simulink model "ROS2"  (R2018b)
settings: Solver=ode5  StartTime=0.0  StopTime=10  FixedStep=0.001  RelTol=1e-3  EnableMultiTasking=on
InitFcn:
  | clear;
  | clc;
  | close all;
  | L1=[1 0 0 -1;-1 1 0 0;0 -1 1 0;0 0 -1 1];
  | 
  | I2=eye(2);
  | LK1=kron(L1,I2);
  | LK1=-LK1;
  | %E matrix
  | E=eye(8);
  | x0=[0 0 0 0 0 0 0 0];
  | x02=[x0(1) x0(3) x0(5) x0(7) x0(2) x0(4) x0(6) x0(8)];
  | x0=x0';
  | 
  | v0=[1 1 2 1 1 1 1 1]';
  | xd=[20 20 30 20 30 10 20 10];
  | 
  | PID=[10,1,0,100];
  | 
  | M=[1 1;1 -1];
StopFcn:
  | figure
  | x_trajectory_1=trajectory(:,1);
  | y_trajectory_1=trajectory(:,5);
  | x_trajectory_2=trajectory(:,2);
  | y_trajectory_2=trajectory(:,6);
  | x_trajectory_3=trajectory(:,3);
  | y_trajectory_3=trajectory(:,7);
  | x_trajectory_4=trajectory(:,4);
  | y_trajectory_4=trajectory(:,8);
  | 
  | plot(x_trajectory_1,y_trajectory_1,x_trajectory_2,y_trajectory_2,x_trajectory_3,y_trajectory_3,x_trajectory_4,y_trajectory_4)
  | 
  | hold on
  | x_path_1=path(:,1);
  | y_path_1=path(:,2);
  | x_path_2=path(:,3);
  | y_path_2=path(:,4);
  | x_path_3=path(:,5);
  | y_path_3=path(:,6);
  | x_path_4=path(:,7);
  | y_path_4=path(:,8);
  | plot(x_path_1,y_path_1,'.',x_path_2,y_path_2,'.',x_path_3,y_path_3,'.',x_path_4,y_path_4,'.')
undefined symbols (not defined in the file): position_real
libraries: simulink x2
settings Model: Creator=108  LastModifiedBy=108
settings OptimizationCC: LifeSpan=inf
settings DebuggingCC: SFUnexpectedBacktrackingDiag=warning  SFNoUnconditionalDefaultTransitionDiag=warning
settings SFSimCC: SimUseLocalCustomCode=off
settings RTWCC: RTWUseLocalCustomCode=off
settings CodeAppCC: StateflowObjectComments=on
settings GRTTargetCC: TargetLangStandard=C89/C90 (ANSI)  GeneratePreprocessorConditionals=Disable all
settings ConfigComp: CovMetricSettings=dw  CovHtmlReporting=on  CovSaveCumulativeToWorkspaceVar=on  CovSaveSingleToWorkspaceVar=on  CovExternalEMLEnable=off

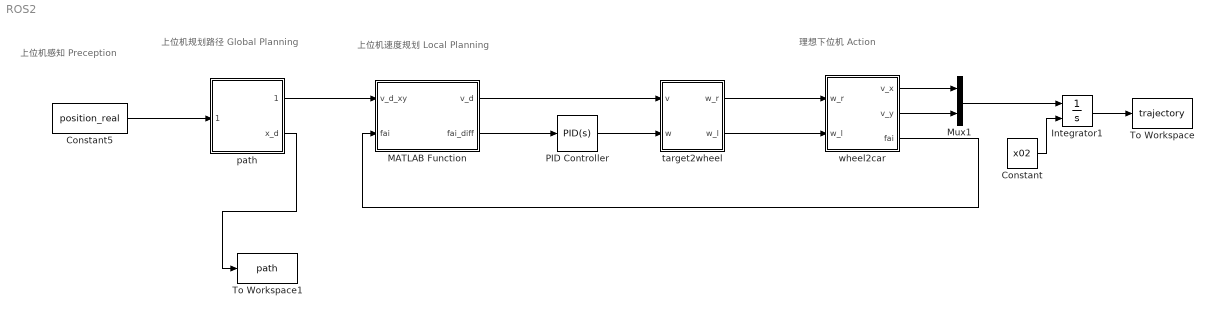
== system ROS2 ==
  note: 上位机速度规划
      | Local Planning
  note: 上位机感知
      | Preception
  note: 理想下位机
      | Action
  note: 上位机规划路径
      | Global Planning
  Constant : Constant  Value=x02
  Constant5 : Constant  Value=position_real
  Integrator1 : Integrator  InitialConditionSource=external
  MATLAB Function : MATLAB Function  TreatAsAtomicUnit=on
  Mux1 : Mux  Inputs=2
  PID Controller : simulink/Continuous/PID Controller  Controller=PID  Form=Parallel  TimeDomain=Continuous-time  SampleTime=-1  IntegratorMethod=Forward Euler  FilterMethod=Forward Euler  ControllerParametersSource=internal  P=200  I=10  D=0  UseFilter=on  N=100  TunerSelectOption=Transfer Function Based (PID Tuner App)  InitialConditionSource=internal  InitialConditionForIntegrator=0  InitialConditionForFilter=0  DifferentiatorICPrevScaledInput=0  ExternalReset=none  TrackingMode=off  Kt=1  LimitOutput=off  UpperSaturationLimit=inf  LowerSaturationLimit=-inf  LinearizeAsGain=on  AntiWindupMode=none  Kb=1  POutMin=[]  POutMax=[]  IOutMin=[]  IOutMax=[]  DOutMin=[]  DOutMax=[]  NOutMin=[]  NOutMax=[]  SumOutMin=[]  SumOutMax=[]  SaturationOutMin=[]  SaturationOutMax=[]  PParamMin=[]  PParamMax=[]  IParamMin=[]  IParamMax=[]  DParamMin=[]  DParamMax=[]  NParamMin=[]  NParamMax=[]  KbParamMin=[]  KbParamMax=[]  KtParamMin=[]  KtParamMax=[]  KbOutMin=[]  KbOutMax=[]  KtOutMin=[]  KtOutMax=[]  IntegratorOutMin=[]  IntegratorOutMax=[]  FilterOutMin=[]  FilterOutMax=[]  SumI1OutMin=[]  SumI1OutMax=[]  SumI2OutMin=[]  SumI2OutMax=[]  SumI3OutMin=[]  SumI3OutMax=[]  SumI4OutMin=[]  SumI4OutMax=[]  SumDOutMin=[]  SumDOutMax=[]  DifferentiatorOutMin=[]  DifferentiatorOutMax=[]  FilterDiffOutCoefMin=[]  FilterDiffOutCoefMax=[]  ReciprocalOutMin=[]  ReciprocalOutMax=[]  SumDenOutMin=[]  SumDenOutMax=[]  SumNumOutMin=[]  SumNumOutMax=[]  DivideOutMin=[]  DivideOutMax=[]  IntegratorContinuousStateAttributes=''  IntegratorStateMustResolveToSignalObject=off  IntegratorRTWStateStorageClass=Auto  FilterContinuousStateAttributes=''  FilterStateMustResolveToSignalObject=off  FilterRTWStateStorageClass=Auto  ParallelPVariant=InternalParameters  IdealPVariant=Disabled  IVariant=InternalParameters  DVariant=InternalParameters  IntegratorVariant=Continuous  SatVariant=Disabled  AWVariant=Passthrough  PCopyVariant=Disabled  TRVariant=Disabled  FdbkBlocksVariant=Forward  IdealPFdbkVariant=Disabled  SatFdbkVariant=Disabled  DerivativeFilterVariant=ContFilter  NVariant=InternalParameters  NCopyVariant=Disabled  FilterICVariant=InternalICsFilter  IntegratorICVariant=InternalICs  ExternalResetVariant=Disabled  TRSumVariant=Passthrough  SumFdbkVariant=Disabled  SumVariant=Sum_PID
  To Workspace : ToWorkspace  VariableName=trajectory  SampleTime=-1
  To Workspace1 : ToWorkspace  VariableName=path  SampleTime=-1
  path : Subsystem
  target2wheel : Subsystem
  wheel2car : Subsystem
  wires:
  target2wheel/1(w_r) -> wheel2car/1(w_r)
  target2wheel/2(w_l) -> wheel2car/2(w_l)
  MATLAB Function/2(fai_diff) -> PID Controller/1
  PID Controller/1 -> target2wheel/2(w)
  wheel2car/3(fai) -> MATLAB Function/2(fai)
  MATLAB Function/1(v_d) -> target2wheel/1(v)
  path/2(x_d) -> To Workspace1/1
  path/1(v_d_xy) -> MATLAB Function/1(v_d_xy)
  Mux1/1 -> Integrator1/1
  Constant/1 -> Integrator1/2
  Integrator1/1 -> To Workspace/1
  wheel2car/1(v_x) -> Mux1/1
  wheel2car/2(v_y) -> Mux1/2
  Constant5/1 -> path/1(position_real)

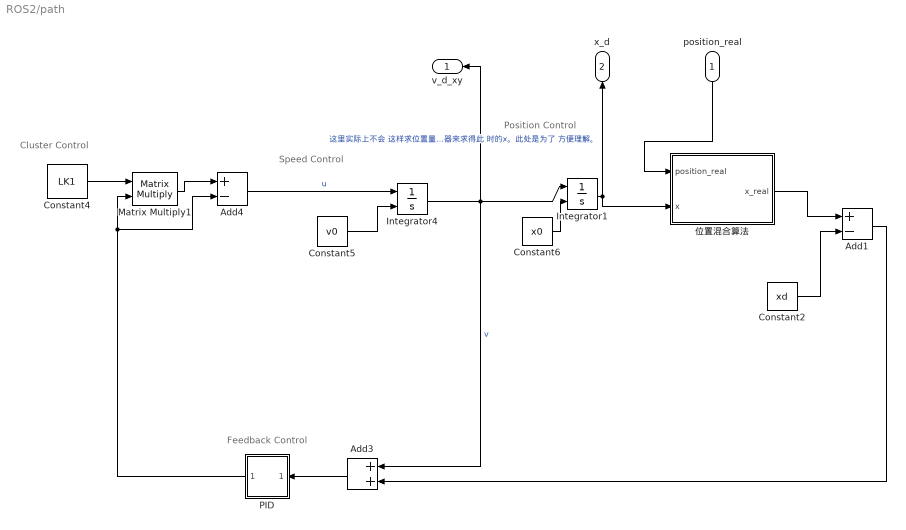
== system ROS2/path ==
  note: Cluster Control
  note: Feedback Control
  note: Position Control
  note: Speed Control
  position_real : Inport
  Add1 : Sum  Inputs=+-
  Add3 : Sum
  Add4 : Sum  Inputs=+-
  Constant2 : Constant  Value=xd
  Constant4 : Constant  Value=LK1
  Constant5 : Constant  Value=v0
  Constant6 : Constant  Value=x0
  Integrator1 : Integrator  InitialConditionSource=external
  Integrator4 : Integrator  InitialConditionSource=external
  Matrix Multiply1 : Product  Multiplication=Matrix(*)
  PID : Subsystem
  位置混合算法 : MATLAB Function  TreatAsAtomicUnit=on
  v_d_xy : Outport
  x_d : Outport  Port=2
  wires:
  Constant4/1 -> Matrix Multiply1/1
  Integrator4/1 -> v_d_xy/1, Integrator1/1, Add3/1  "v"
  Add4/1 -> Integrator4/1  "u"
  Matrix Multiply1/1 -> Add4/1
  PID/1(Out1) -> Matrix Multiply1/2, Add4/2
  Add1/1 -> Add3/2
  Add3/1 -> PID/1(In1)
  Integrator1/1 -> x_d/1, 位置混合算法/2(x)  "这里实际上不会 这样求位置量， 因为很不准确， 而是会直接通过 编码器来求得此 时的x。此处是为了 方便理解。"
  Constant2/1 -> Add1/2
  Constant5/1 -> Integrator4/2
  Constant6/1 -> Integrator1/2
  position_real/1 -> 位置混合算法/1(position_real)
  位置混合算法/1(x_real) -> Add1/1

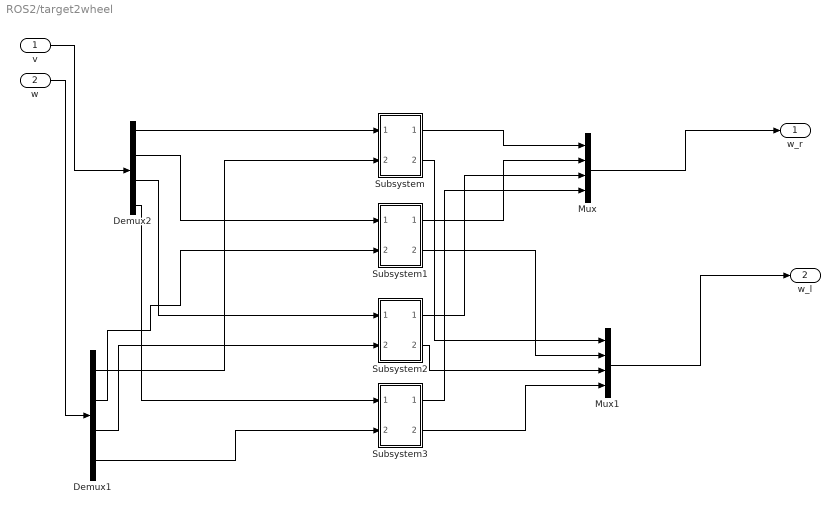
== system ROS2/target2wheel ==
  v : Inport
  w : Inport  Port=2
  Demux1 : Demux
  Demux2 : Demux
  Mux : Mux
  Mux1 : Mux
  Subsystem : Subsystem
  Subsystem1 : Subsystem
  Subsystem2 : Subsystem
  Subsystem3 : Subsystem
  w_r : Outport
  w_l : Outport  Port=2
  wires:
  v/1 -> Demux2/1
  w/1 -> Demux1/1
  Demux2/2 -> Subsystem1/1(In1)
  Demux2/3 -> Subsystem2/1(In1)
  Demux2/4 -> Subsystem3/1(In1)
  Demux1/2 -> Subsystem1/2(In2)
  Demux1/3 -> Subsystem2/2(In2)
  Demux1/4 -> Subsystem3/2(In2)
  Demux2/1 -> Subsystem/1(In1)
  Demux1/1 -> Subsystem/2(In2)
  Subsystem/1(Out1) -> Mux/1
  Subsystem1/1(Out1) -> Mux/2
  Subsystem2/1(Out1) -> Mux/3
  Subsystem3/1(Out1) -> Mux/4
  Subsystem/2(Out2) -> Mux1/1
  Subsystem1/2(Out2) -> Mux1/2
  Subsystem2/2(Out2) -> Mux1/3
  Subsystem3/2(Out2) -> Mux1/4
  Mux/1 -> w_r/1
  Mux1/1 -> w_l/1

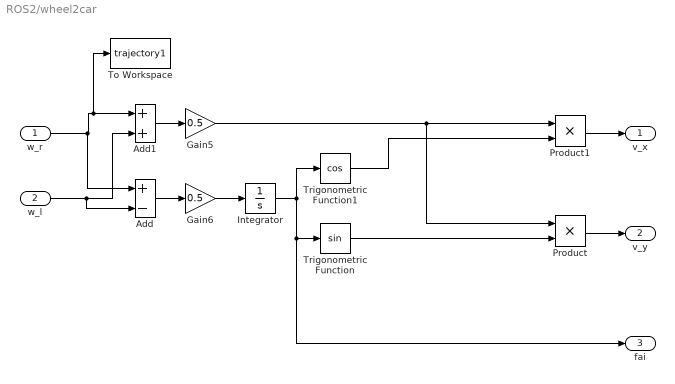
== system ROS2/wheel2car ==
  w_r : Inport
  w_l : Inport  Port=2
  Add : Sum  Inputs=+-
  Add1 : Sum
  Gain5 : Gain  Gain=0.5
  Gain6 : Gain  Gain=0.5
  Integrator : Integrator
  Product : Product
  Product1 : Product
  To Workspace : ToWorkspace  VariableName=trajectory1  SampleTime=-1
  Trigonometric Function : Trigonometry
  Trigonometric Function1 : Trigonometry  Operator=cos
  v_x : Outport
  v_y : Outport  Port=2
  fai : Outport  Port=3
  wires:
  Gain5/1 -> Product1/1, Product/1
  Gain6/1 -> Integrator/1
  Integrator/1 -> Trigonometric Function1/1, fai/1, Trigonometric Function/1
  Trigonometric Function/1 -> Product/2
  Trigonometric Function1/1 -> Product1/2
  w_r/1 -> Add/1, To Workspace/1, Add1/1
  w_l/1 -> Add/2, Add1/2
  Add1/1 -> Gain5/1
  Add/1 -> Gain6/1
  Product1/1 -> v_x/1
  Product/1 -> v_y/1

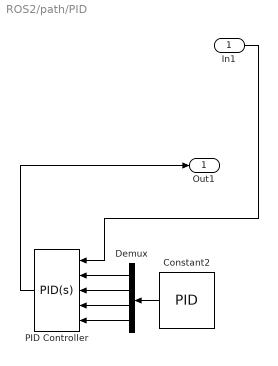
== system ROS2/path/PID ==
  In1 : Inport
  Constant2 : Constant  Value=PID
  Demux : Demux
  PID Controller : simulink/Continuous/PID Controller  Controller=PID  Form=Parallel  TimeDomain=Continuous-time  SampleTime=-1  IntegratorMethod=Forward Euler  FilterMethod=Forward Euler  ControllerParametersSource=external  P=30  I=1  D=0  UseFilter=on  N=100  TunerSelectOption=Transfer Function Based (PID Tuner App)  InitialConditionSource=internal  InitialConditionForIntegrator=0  InitialConditionForFilter=0  DifferentiatorICPrevScaledInput=0  ExternalReset=none  TrackingMode=off  Kt=1  LimitOutput=off  UpperSaturationLimit=inf  LowerSaturationLimit=-inf  LinearizeAsGain=on  AntiWindupMode=none  Kb=1  POutMin=[]  POutMax=[]  IOutMin=[]  IOutMax=[]  DOutMin=[]  DOutMax=[]  NOutMin=[]  NOutMax=[]  SumOutMin=[]  SumOutMax=[]  SaturationOutMin=[]  SaturationOutMax=[]  PParamMin=[]  PParamMax=[]  IParamMin=[]  IParamMax=[]  DParamMin=[]  DParamMax=[]  NParamMin=[]  NParamMax=[]  KbParamMin=[]  KbParamMax=[]  KtParamMin=[]  KtParamMax=[]  KbOutMin=[]  KbOutMax=[]  KtOutMin=[]  KtOutMax=[]  IntegratorOutMin=[]  IntegratorOutMax=[]  FilterOutMin=[]  FilterOutMax=[]  SumI1OutMin=[]  SumI1OutMax=[]  SumI2OutMin=[]  SumI2OutMax=[]  SumI3OutMin=[]  SumI3OutMax=[]  SumI4OutMin=[]  SumI4OutMax=[]  SumDOutMin=[]  SumDOutMax=[]  DifferentiatorOutMin=[]  DifferentiatorOutMax=[]  FilterDiffOutCoefMin=[]  FilterDiffOutCoefMax=[]  ReciprocalOutMin=[]  ReciprocalOutMax=[]  SumDenOutMin=[]  SumDenOutMax=[]  SumNumOutMin=[]  SumNumOutMax=[]  DivideOutMin=[]  DivideOutMax=[]  IntegratorContinuousStateAttributes=''  IntegratorStateMustResolveToSignalObject=off  IntegratorRTWStateStorageClass=Auto  FilterContinuousStateAttributes=''  FilterStateMustResolveToSignalObject=off  FilterRTWStateStorageClass=Auto  ParallelPVariant=ExternalParameters  IdealPVariant=Disabled  IVariant=ExternalParameters  DVariant=ExternalParameters  IntegratorVariant=Continuous  SatVariant=Disabled  AWVariant=Passthrough  PCopyVariant=Disabled  TRVariant=Disabled  FdbkBlocksVariant=Forward  IdealPFdbkVariant=Disabled  SatFdbkVariant=Disabled  DerivativeFilterVariant=ContFilter  NVariant=ExternalParameters  NCopyVariant=Disabled  FilterICVariant=InternalICsFilter  IntegratorICVariant=InternalICs  ExternalResetVariant=Disabled  TRSumVariant=Passthrough  SumFdbkVariant=Disabled  SumVariant=Sum_PID
  Out1 : Outport
  wires:
  Demux/4 -> PID Controller/5
  Demux/3 -> PID Controller/4
  Demux/2 -> PID Controller/3
  Demux/1 -> PID Controller/2
  Constant2/1 -> Demux/1
  In1/1 -> PID Controller/1
  PID Controller/1 -> Out1/1

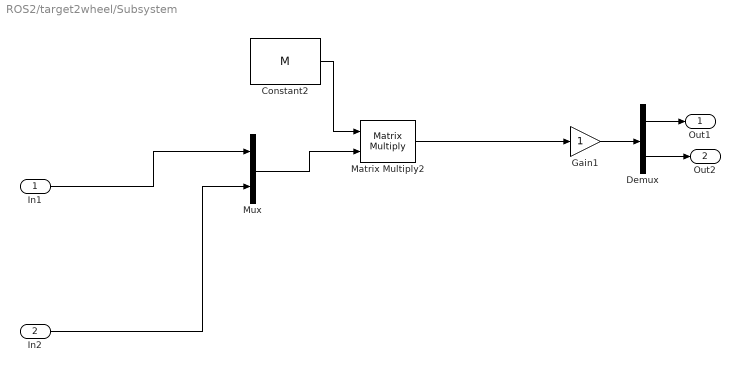
== system ROS2/target2wheel/Subsystem ==
  In1 : Inport
  In2 : Inport  Port=2
  Constant2 : Constant  Value=M
  Demux : Demux  Outputs=2
  Gain1 : Gain
  Matrix Multiply2 : Product  Multiplication=Matrix(*)
  Mux : Mux  Inputs=2
  Out1 : Outport
  Out2 : Outport  Port=2
  wires:
  Demux/1 -> Out1/1
  In2/1 -> Mux/2
  Mux/1 -> Matrix Multiply2/2
  Gain1/1 -> Demux/1
  In1/1 -> Mux/1
  Matrix Multiply2/1 -> Gain1/1
  Constant2/1 -> Matrix Multiply2/1
  Demux/2 -> Out2/1

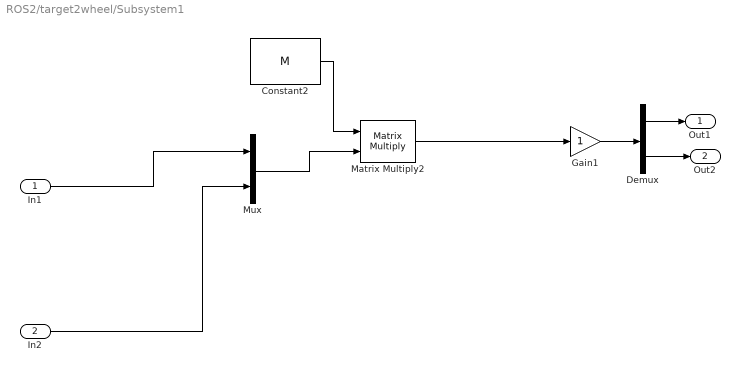
== system ROS2/target2wheel/Subsystem1 ==
  In1 : Inport
  In2 : Inport  Port=2
  Constant2 : Constant  Value=M
  Demux : Demux  Outputs=2
  Gain1 : Gain
  Matrix Multiply2 : Product  Multiplication=Matrix(*)
  Mux : Mux  Inputs=2
  Out1 : Outport
  Out2 : Outport  Port=2
  wires:
  Demux/2 -> Out2/1
  Constant2/1 -> Matrix Multiply2/1
  Matrix Multiply2/1 -> Gain1/1
  In1/1 -> Mux/1
  Gain1/1 -> Demux/1
  Mux/1 -> Matrix Multiply2/2
  In2/1 -> Mux/2
  Demux/1 -> Out1/1

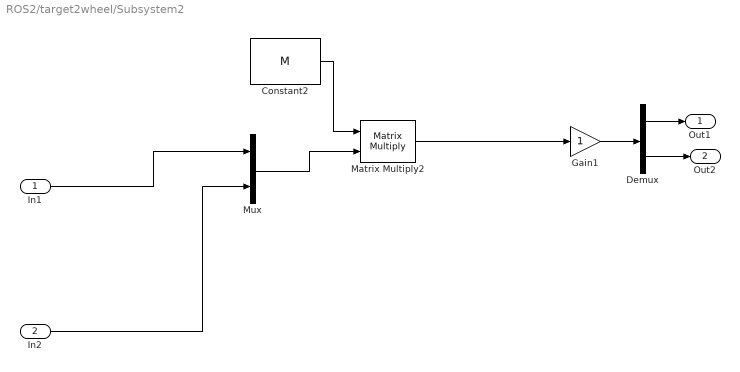
== system ROS2/target2wheel/Subsystem2 ==
  In1 : Inport
  In2 : Inport  Port=2
  Constant2 : Constant  Value=M
  Demux : Demux  Outputs=2
  Gain1 : Gain
  Matrix Multiply2 : Product  Multiplication=Matrix(*)
  Mux : Mux  Inputs=2
  Out1 : Outport
  Out2 : Outport  Port=2
  wires:
  Demux/1 -> Out1/1
  In2/1 -> Mux/2
  Mux/1 -> Matrix Multiply2/2
  Gain1/1 -> Demux/1
  In1/1 -> Mux/1
  Matrix Multiply2/1 -> Gain1/1
  Constant2/1 -> Matrix Multiply2/1
  Demux/2 -> Out2/1

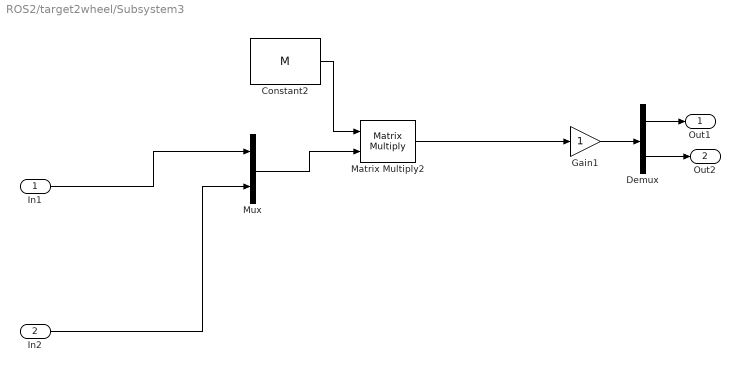
== system ROS2/target2wheel/Subsystem3 ==
  In1 : Inport
  In2 : Inport  Port=2
  Constant2 : Constant  Value=M
  Demux : Demux  Outputs=2
  Gain1 : Gain
  Matrix Multiply2 : Product  Multiplication=Matrix(*)
  Mux : Mux  Inputs=2
  Out1 : Outport
  Out2 : Outport  Port=2
  wires:
  Demux/2 -> Out2/1
  Constant2/1 -> Matrix Multiply2/1
  Matrix Multiply2/1 -> Gain1/1
  In1/1 -> Mux/1
  Gain1/1 -> Demux/1
  Mux/1 -> Matrix Multiply2/2
  In2/1 -> Mux/2
  Demux/1 -> Out1/1

== matlab function ROS2/path/位置混合算法 ==
  data: position_real input; x_real output; x input
function x_real = fcn(position_real,x)
%#codegen
position_real=0;
x_real=x;
end

== matlab function ROS2/MATLAB Function ==
  data: v_d_xy input; v_d output; fai_diff output; fai input
function [v_d,fai_diff]  = fcn(v_d_xy,fai)
%#codegen

%v_d=[0];
%fai_diff=[0];
v_d=[0 0 0 0];
fai_diff=[0 0 0 0];
fai_d=[0 0 0 0];
j=1;

for i=1:2:7
    v_d(j) = sqrt(v_d_xy(i).^2+ v_d_xy(i+1).^2);
    fai_d(j) = atan2(v_d_xy(i+1),v_d_xy(i));
    fai_diff(j)= fai_d(j)-fai(j);
    if fai_diff(j)>pi
        fai_diff(j)=fai_diff(j)-2*pi*round(fai_diff(j)/(2*pi));
    elseif fai_diff(j)<-pi
        fai_diff(j)=fai_diff(j)+2*pi*round(fai_diff(j)/(-2*pi));      
    end
   
   j=j+1;
end

end
